simulink model "MIL_Simulation_Position_Control"  (R2023a)
settings: Solver=VariableStepAuto  StartTime=0.0  StopTime=18  RelTol=1e-3
undefined symbols (not defined in the file): Ad, Bd, Cd, Dd, Ts
settings Model: Creator=Marco  LastModifiedBy=Marco

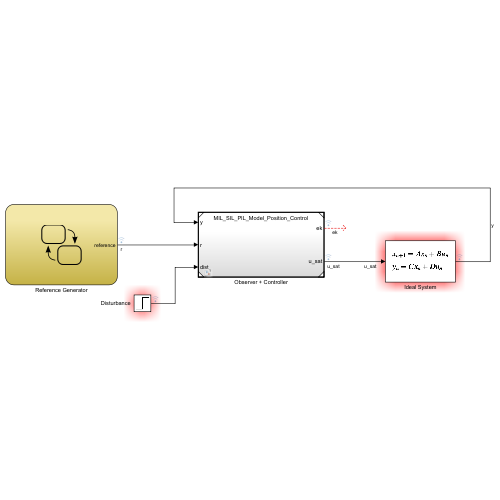
[thumbnail: Simulink's stored preview of the top-level diagram]
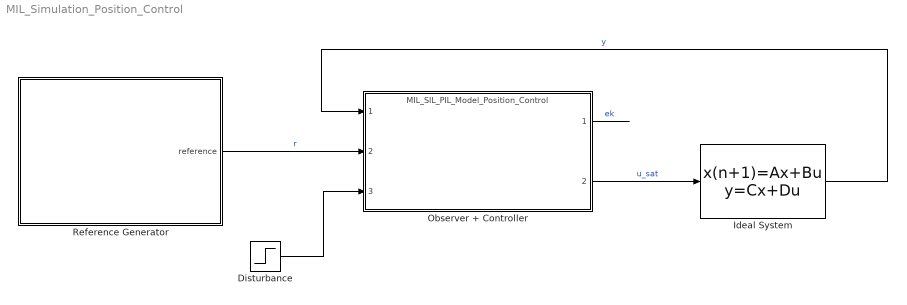
== system MIL_Simulation_Position_Control ==
  Disturbance : Step  Time=3  After=1.2  SampleTime=Ts
  Ideal System : DiscreteStateSpace  A=Ad  B=Bd  C=Cd  D=Dd  SampleTime=Ts
  Observer + Controller : ModelReference  ModelNameDialog=MIL_SIL_PIL_Model_Position_Control.slx  SimulationMode=Normal  ModelReferenceVersion=1.9
  Reference Generator : Stateflow chart  TreatAsAtomicUnit=on
  wires:
  Reference Generator/1(reference) -> Observer + Controller/2  "r"
  Ideal System/1 -> Observer + Controller/1  "y"
  Observer + Controller/1 -> ?  "ek"
  Observer + Controller/2 -> Ideal System/1  "u_sat"
  Disturbance/1 -> Observer + Controller/3

== stateflow chart MIL_Simulation_Position_Control/Reference Generator ==
  state Start
    reference = 0;
  state State1
    reference = deg2rad(30)
  state State4
    reference = deg2rad(-30)
  state State2
    reference = deg2rad(180)
  state State3
    reference = deg2rad(-180)
  state State5
    reference = 0
  (default) -> Start
  Start -> State1 : [after(3,sec)]
  State1 -> State4 : [after(3, sec)]
  State4 -> State2 : [after(3,sec)]
  State3 -> Start : [after(3,sec)]
  State2 -> State5 : [after(3,sec)]
  State5 -> State3 : [after(3,sec)]
  data: reference output
